simulink model "testManyDelay"  (Simulink 7.4)
settings: Solver=ode45  StartTime=0.0  StopTime=10.0  RelTol=1e-3
libraries: BLOM_Lib x1
settings Model: Creator=Eric  LastModifiedBy=Eric

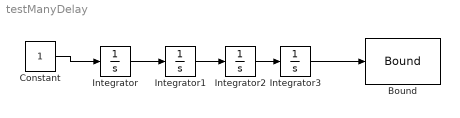
== system testManyDelay ==
  Bound : BLOM_Lib/Bound  SystemSampleTime=-1  ub=1  lb=0  initial_step=on  final_step=on  intermediate_step=on
  Constant : Constant  OutDataType=fixdt(1, 16)  OutScaling=2^0
  Integrator{,1..3} (4 alike) : Integrator
  wires:
  Constant/1 -> Integrator/1
  Integrator/1 -> Integrator1/1
  Integrator1/1 -> Integrator2/1
  Integrator2/1 -> Integrator3/1
  Integrator3/1 -> Bound/1
